simulink model "ex_5_3"  (R2020b)
settings: Solver=VariableStepAuto  StartTime=0.0  StopTime=10.0  RelTol=1e-3
settings Model: Creator=duzun  LastModifiedBy=duzun

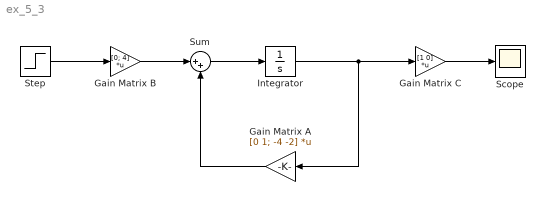
== system ex_5_3 ==
  Gain Matrix A : Gain  Gain=[0 1; -4 -2]  Multiplication=Matrix(K*u)
  Gain Matrix B : Gain  Gain=[0; 4]  Multiplication=Matrix(K*u)
  Gain Matrix C : Gain  Gain=[1 0]  Multiplication=Matrix(K*u)
  Integrator : Integrator
  Scope : Scope
  Step : Step  Time=0  SampleTime=0
  Sum : Sum  Inputs=|++
  wires:
  Gain Matrix C/1 -> Scope/1
  Sum/1 -> Integrator/1
  Integrator/1 -> Gain Matrix A/1, Gain Matrix C/1
  Step/1 -> Gain Matrix B/1
  Gain Matrix B/1 -> Sum/1
  Gain Matrix A/1 -> Sum/2
